simulink library "speedgoatlib_mscp"  (R2024b)
settings: Solver=VariableStepAuto  StartTime=0.0  StopTime=10.0  RelTol=1e-3
libraries: slrealtimeethercatlib x517, simulink x316, hdlsllib x168, $bdroot x11, slrealtimeutilitieslib x1
(part 4 of 5)

== system speedgoatlib_mscp/Templates/MSCP SC2191 Read Advanced Template/Channel_07 ==
  Bus Creator : BusCreator  Inputs=6  OutDataTypeStr=Bus: MscpBus_SC2191_Channel_Advanced_Read
      settings: InheritFromInputs=off
  Vhigh : slrealtimeethercatlib/EtherCAT PDO Receive  Priority=2  sig_name=Uninitialized Block  sig_offset=144  sig_type=uint8  type_size=8  sig_dim=1  device_id=0  sample_time=0.010000
  Vhigh_Gain : slrealtimeethercatlib/EtherCAT PDO Receive  Priority=2  sig_name=Uninitialized Block  sig_offset=144  sig_type=uint8  type_size=8  sig_dim=1  device_id=0  sample_time=0.010000
  Vhigh_Offset : slrealtimeethercatlib/EtherCAT PDO Receive  Priority=2  sig_name=Uninitialized Block  sig_offset=144  sig_type=uint8  type_size=8  sig_dim=1  device_id=0  sample_time=0.010000
  Vlow : slrealtimeethercatlib/EtherCAT PDO Receive  Priority=2  sig_name=Uninitialized Block  sig_offset=144  sig_type=uint8  type_size=8  sig_dim=1  device_id=0  sample_time=0.010000
  Vlow_Gain : slrealtimeethercatlib/EtherCAT PDO Receive  Priority=2  sig_name=Uninitialized Block  sig_offset=144  sig_type=uint8  type_size=8  sig_dim=1  device_id=0  sample_time=0.010000
  Vlow_Offset : slrealtimeethercatlib/EtherCAT PDO Receive  Priority=2  sig_name=Uninitialized Block  sig_offset=144  sig_type=uint8  type_size=8  sig_dim=1  device_id=0  sample_time=0.010000
  Out1 : Outport
  wires:
  Vhigh/1 -> Bus Creator/2
  Vlow/1 -> Bus Creator/1
  Bus Creator/1 -> Out1/1
  Vlow_Offset/1 -> Bus Creator/3
  Vlow_Gain/1 -> Bus Creator/4
  Vhigh_Offset/1 -> Bus Creator/5
  Vhigh_Gain/1 -> Bus Creator/6

== system speedgoatlib_mscp/Templates/MSCP SC2191 Read Advanced Template/Channel_08 ==
  Bus Creator : BusCreator  Inputs=6  OutDataTypeStr=Bus: MscpBus_SC2191_Channel_Advanced_Read
      settings: InheritFromInputs=off
  Vhigh : slrealtimeethercatlib/EtherCAT PDO Receive  Priority=2  sig_name=Uninitialized Block  sig_offset=144  sig_type=uint8  type_size=8  sig_dim=1  device_id=0  sample_time=0.010000
  Vhigh_Gain : slrealtimeethercatlib/EtherCAT PDO Receive  Priority=2  sig_name=Uninitialized Block  sig_offset=144  sig_type=uint8  type_size=8  sig_dim=1  device_id=0  sample_time=0.010000
  Vhigh_Offset : slrealtimeethercatlib/EtherCAT PDO Receive  Priority=2  sig_name=Uninitialized Block  sig_offset=144  sig_type=uint8  type_size=8  sig_dim=1  device_id=0  sample_time=0.010000
  Vlow : slrealtimeethercatlib/EtherCAT PDO Receive  Priority=2  sig_name=Uninitialized Block  sig_offset=144  sig_type=uint8  type_size=8  sig_dim=1  device_id=0  sample_time=0.010000
  Vlow_Gain : slrealtimeethercatlib/EtherCAT PDO Receive  Priority=2  sig_name=Uninitialized Block  sig_offset=144  sig_type=uint8  type_size=8  sig_dim=1  device_id=0  sample_time=0.010000
  Vlow_Offset : slrealtimeethercatlib/EtherCAT PDO Receive  Priority=2  sig_name=Uninitialized Block  sig_offset=144  sig_type=uint8  type_size=8  sig_dim=1  device_id=0  sample_time=0.010000
  Out1 : Outport
  wires:
  Vhigh_Gain/1 -> Bus Creator/6
  Vhigh_Offset/1 -> Bus Creator/5
  Vlow_Gain/1 -> Bus Creator/4
  Vlow_Offset/1 -> Bus Creator/3
  Bus Creator/1 -> Out1/1
  Vlow/1 -> Bus Creator/1
  Vhigh/1 -> Bus Creator/2

== system speedgoatlib_mscp/Templates/MSCP SC2191 Read Advanced Template/Channel_09 ==
  Bus Creator : BusCreator  Inputs=6  OutDataTypeStr=Bus: MscpBus_SC2191_Channel_Advanced_Read
      settings: InheritFromInputs=off
  Vhigh : slrealtimeethercatlib/EtherCAT PDO Receive  Priority=2  sig_name=Uninitialized Block  sig_offset=144  sig_type=uint8  type_size=8  sig_dim=1  device_id=0  sample_time=0.010000
  Vhigh_Gain : slrealtimeethercatlib/EtherCAT PDO Receive  Priority=2  sig_name=Uninitialized Block  sig_offset=144  sig_type=uint8  type_size=8  sig_dim=1  device_id=0  sample_time=0.010000
  Vhigh_Offset : slrealtimeethercatlib/EtherCAT PDO Receive  Priority=2  sig_name=Uninitialized Block  sig_offset=144  sig_type=uint8  type_size=8  sig_dim=1  device_id=0  sample_time=0.010000
  Vlow : slrealtimeethercatlib/EtherCAT PDO Receive  Priority=2  sig_name=Uninitialized Block  sig_offset=144  sig_type=uint8  type_size=8  sig_dim=1  device_id=0  sample_time=0.010000
  Vlow_Gain : slrealtimeethercatlib/EtherCAT PDO Receive  Priority=2  sig_name=Uninitialized Block  sig_offset=144  sig_type=uint8  type_size=8  sig_dim=1  device_id=0  sample_time=0.010000
  Vlow_Offset : slrealtimeethercatlib/EtherCAT PDO Receive  Priority=2  sig_name=Uninitialized Block  sig_offset=144  sig_type=uint8  type_size=8  sig_dim=1  device_id=0  sample_time=0.010000
  Out1 : Outport
  wires:
  Vhigh/1 -> Bus Creator/2
  Vlow/1 -> Bus Creator/1
  Bus Creator/1 -> Out1/1
  Vlow_Offset/1 -> Bus Creator/3
  Vlow_Gain/1 -> Bus Creator/4
  Vhigh_Offset/1 -> Bus Creator/5
  Vhigh_Gain/1 -> Bus Creator/6

== system speedgoatlib_mscp/Templates/MSCP SC2191 Read Advanced Template/Channel_10 ==
  Bus Creator : BusCreator  Inputs=6  OutDataTypeStr=Bus: MscpBus_SC2191_Channel_Advanced_Read
      settings: InheritFromInputs=off
  Vhigh : slrealtimeethercatlib/EtherCAT PDO Receive  Priority=2  sig_name=Uninitialized Block  sig_offset=144  sig_type=uint8  type_size=8  sig_dim=1  device_id=0  sample_time=0.010000
  Vhigh_Gain : slrealtimeethercatlib/EtherCAT PDO Receive  Priority=2  sig_name=Uninitialized Block  sig_offset=144  sig_type=uint8  type_size=8  sig_dim=1  device_id=0  sample_time=0.010000
  Vhigh_Offset : slrealtimeethercatlib/EtherCAT PDO Receive  Priority=2  sig_name=Uninitialized Block  sig_offset=144  sig_type=uint8  type_size=8  sig_dim=1  device_id=0  sample_time=0.010000
  Vlow : slrealtimeethercatlib/EtherCAT PDO Receive  Priority=2  sig_name=Uninitialized Block  sig_offset=144  sig_type=uint8  type_size=8  sig_dim=1  device_id=0  sample_time=0.010000
  Vlow_Gain : slrealtimeethercatlib/EtherCAT PDO Receive  Priority=2  sig_name=Uninitialized Block  sig_offset=144  sig_type=uint8  type_size=8  sig_dim=1  device_id=0  sample_time=0.010000
  Vlow_Offset : slrealtimeethercatlib/EtherCAT PDO Receive  Priority=2  sig_name=Uninitialized Block  sig_offset=144  sig_type=uint8  type_size=8  sig_dim=1  device_id=0  sample_time=0.010000
  Out1 : Outport
  wires:
  Vhigh_Gain/1 -> Bus Creator/6
  Vhigh_Offset/1 -> Bus Creator/5
  Vlow_Gain/1 -> Bus Creator/4
  Vlow_Offset/1 -> Bus Creator/3
  Bus Creator/1 -> Out1/1
  Vlow/1 -> Bus Creator/1
  Vhigh/1 -> Bus Creator/2

== system speedgoatlib_mscp/Templates/MSCP SC2191 Read Advanced Template/Channel_11 ==
  Bus Creator : BusCreator  Inputs=6  OutDataTypeStr=Bus: MscpBus_SC2191_Channel_Advanced_Read
      settings: InheritFromInputs=off
  Vhigh : slrealtimeethercatlib/EtherCAT PDO Receive  Priority=2  sig_name=Uninitialized Block  sig_offset=144  sig_type=uint8  type_size=8  sig_dim=1  device_id=0  sample_time=0.010000
  Vhigh_Gain : slrealtimeethercatlib/EtherCAT PDO Receive  Priority=2  sig_name=Uninitialized Block  sig_offset=144  sig_type=uint8  type_size=8  sig_dim=1  device_id=0  sample_time=0.010000
  Vhigh_Offset : slrealtimeethercatlib/EtherCAT PDO Receive  Priority=2  sig_name=Uninitialized Block  sig_offset=144  sig_type=uint8  type_size=8  sig_dim=1  device_id=0  sample_time=0.010000
  Vlow : slrealtimeethercatlib/EtherCAT PDO Receive  Priority=2  sig_name=Uninitialized Block  sig_offset=144  sig_type=uint8  type_size=8  sig_dim=1  device_id=0  sample_time=0.010000
  Vlow_Gain : slrealtimeethercatlib/EtherCAT PDO Receive  Priority=2  sig_name=Uninitialized Block  sig_offset=144  sig_type=uint8  type_size=8  sig_dim=1  device_id=0  sample_time=0.010000
  Vlow_Offset : slrealtimeethercatlib/EtherCAT PDO Receive  Priority=2  sig_name=Uninitialized Block  sig_offset=144  sig_type=uint8  type_size=8  sig_dim=1  device_id=0  sample_time=0.010000
  Out1 : Outport
  wires:
  Vhigh/1 -> Bus Creator/2
  Vlow/1 -> Bus Creator/1
  Bus Creator/1 -> Out1/1
  Vlow_Offset/1 -> Bus Creator/3
  Vlow_Gain/1 -> Bus Creator/4
  Vhigh_Offset/1 -> Bus Creator/5
  Vhigh_Gain/1 -> Bus Creator/6

== system speedgoatlib_mscp/Templates/MSCP SC2191 Read Advanced Template/Channel_12 ==
  Bus Creator : BusCreator  Inputs=6  OutDataTypeStr=Bus: MscpBus_SC2191_Channel_Advanced_Read
      settings: InheritFromInputs=off
  Vhigh : slrealtimeethercatlib/EtherCAT PDO Receive  Priority=2  sig_name=Uninitialized Block  sig_offset=144  sig_type=uint8  type_size=8  sig_dim=1  device_id=0  sample_time=0.010000
  Vhigh_Gain : slrealtimeethercatlib/EtherCAT PDO Receive  Priority=2  sig_name=Uninitialized Block  sig_offset=144  sig_type=uint8  type_size=8  sig_dim=1  device_id=0  sample_time=0.010000
  Vhigh_Offset : slrealtimeethercatlib/EtherCAT PDO Receive  Priority=2  sig_name=Uninitialized Block  sig_offset=144  sig_type=uint8  type_size=8  sig_dim=1  device_id=0  sample_time=0.010000
  Vlow : slrealtimeethercatlib/EtherCAT PDO Receive  Priority=2  sig_name=Uninitialized Block  sig_offset=144  sig_type=uint8  type_size=8  sig_dim=1  device_id=0  sample_time=0.010000
  Vlow_Gain : slrealtimeethercatlib/EtherCAT PDO Receive  Priority=2  sig_name=Uninitialized Block  sig_offset=144  sig_type=uint8  type_size=8  sig_dim=1  device_id=0  sample_time=0.010000
  Vlow_Offset : slrealtimeethercatlib/EtherCAT PDO Receive  Priority=2  sig_name=Uninitialized Block  sig_offset=144  sig_type=uint8  type_size=8  sig_dim=1  device_id=0  sample_time=0.010000
  Out1 : Outport
  wires:
  Vhigh_Gain/1 -> Bus Creator/6
  Vhigh_Offset/1 -> Bus Creator/5
  Vlow_Gain/1 -> Bus Creator/4
  Vlow_Offset/1 -> Bus Creator/3
  Bus Creator/1 -> Out1/1
  Vlow/1 -> Bus Creator/1
  Vhigh/1 -> Bus Creator/2

== system speedgoatlib_mscp/Templates/MSCP SC2191 Read Advanced Template/Channel_13 ==
  Bus Creator : BusCreator  Inputs=6  OutDataTypeStr=Bus: MscpBus_SC2191_Channel_Advanced_Read
      settings: InheritFromInputs=off
  Vhigh : slrealtimeethercatlib/EtherCAT PDO Receive  Priority=2  sig_name=Uninitialized Block  sig_offset=144  sig_type=uint8  type_size=8  sig_dim=1  device_id=0  sample_time=0.010000
  Vhigh_Gain : slrealtimeethercatlib/EtherCAT PDO Receive  Priority=2  sig_name=Uninitialized Block  sig_offset=144  sig_type=uint8  type_size=8  sig_dim=1  device_id=0  sample_time=0.010000
  Vhigh_Offset : slrealtimeethercatlib/EtherCAT PDO Receive  Priority=2  sig_name=Uninitialized Block  sig_offset=144  sig_type=uint8  type_size=8  sig_dim=1  device_id=0  sample_time=0.010000
  Vlow : slrealtimeethercatlib/EtherCAT PDO Receive  Priority=2  sig_name=Uninitialized Block  sig_offset=144  sig_type=uint8  type_size=8  sig_dim=1  device_id=0  sample_time=0.010000
  Vlow_Gain : slrealtimeethercatlib/EtherCAT PDO Receive  Priority=2  sig_name=Uninitialized Block  sig_offset=144  sig_type=uint8  type_size=8  sig_dim=1  device_id=0  sample_time=0.010000
  Vlow_Offset : slrealtimeethercatlib/EtherCAT PDO Receive  Priority=2  sig_name=Uninitialized Block  sig_offset=144  sig_type=uint8  type_size=8  sig_dim=1  device_id=0  sample_time=0.010000
  Out1 : Outport
  wires:
  Vhigh/1 -> Bus Creator/2
  Vlow/1 -> Bus Creator/1
  Bus Creator/1 -> Out1/1
  Vlow_Offset/1 -> Bus Creator/3
  Vlow_Gain/1 -> Bus Creator/4
  Vhigh_Offset/1 -> Bus Creator/5
  Vhigh_Gain/1 -> Bus Creator/6

== system speedgoatlib_mscp/Templates/MSCP SC2191 Read Advanced Template/Channel_14 ==
  Bus Creator : BusCreator  Inputs=6  OutDataTypeStr=Bus: MscpBus_SC2191_Channel_Advanced_Read
      settings: InheritFromInputs=off
  Vhigh : slrealtimeethercatlib/EtherCAT PDO Receive  Priority=2  sig_name=Uninitialized Block  sig_offset=144  sig_type=uint8  type_size=8  sig_dim=1  device_id=0  sample_time=0.010000
  Vhigh_Gain : slrealtimeethercatlib/EtherCAT PDO Receive  Priority=2  sig_name=Uninitialized Block  sig_offset=144  sig_type=uint8  type_size=8  sig_dim=1  device_id=0  sample_time=0.010000
  Vhigh_Offset : slrealtimeethercatlib/EtherCAT PDO Receive  Priority=2  sig_name=Uninitialized Block  sig_offset=144  sig_type=uint8  type_size=8  sig_dim=1  device_id=0  sample_time=0.010000
  Vlow : slrealtimeethercatlib/EtherCAT PDO Receive  Priority=2  sig_name=Uninitialized Block  sig_offset=144  sig_type=uint8  type_size=8  sig_dim=1  device_id=0  sample_time=0.010000
  Vlow_Gain : slrealtimeethercatlib/EtherCAT PDO Receive  Priority=2  sig_name=Uninitialized Block  sig_offset=144  sig_type=uint8  type_size=8  sig_dim=1  device_id=0  sample_time=0.010000
  Vlow_Offset : slrealtimeethercatlib/EtherCAT PDO Receive  Priority=2  sig_name=Uninitialized Block  sig_offset=144  sig_type=uint8  type_size=8  sig_dim=1  device_id=0  sample_time=0.010000
  Out1 : Outport
  wires:
  Vhigh_Gain/1 -> Bus Creator/6
  Vhigh_Offset/1 -> Bus Creator/5
  Vlow_Gain/1 -> Bus Creator/4
  Vlow_Offset/1 -> Bus Creator/3
  Bus Creator/1 -> Out1/1
  Vlow/1 -> Bus Creator/1
  Vhigh/1 -> Bus Creator/2

== system speedgoatlib_mscp/Templates/MSCP SC2191 Read Advanced Template/Channel_15 ==
  Bus Creator : BusCreator  Inputs=6  OutDataTypeStr=Bus: MscpBus_SC2191_Channel_Advanced_Read
      settings: InheritFromInputs=off
  Vhigh : slrealtimeethercatlib/EtherCAT PDO Receive  Priority=2  sig_name=Uninitialized Block  sig_offset=144  sig_type=uint8  type_size=8  sig_dim=1  device_id=0  sample_time=0.010000
  Vhigh_Gain : slrealtimeethercatlib/EtherCAT PDO Receive  Priority=2  sig_name=Uninitialized Block  sig_offset=144  sig_type=uint8  type_size=8  sig_dim=1  device_id=0  sample_time=0.010000
  Vhigh_Offset : slrealtimeethercatlib/EtherCAT PDO Receive  Priority=2  sig_name=Uninitialized Block  sig_offset=144  sig_type=uint8  type_size=8  sig_dim=1  device_id=0  sample_time=0.010000
  Vlow : slrealtimeethercatlib/EtherCAT PDO Receive  Priority=2  sig_name=Uninitialized Block  sig_offset=144  sig_type=uint8  type_size=8  sig_dim=1  device_id=0  sample_time=0.010000
  Vlow_Gain : slrealtimeethercatlib/EtherCAT PDO Receive  Priority=2  sig_name=Uninitialized Block  sig_offset=144  sig_type=uint8  type_size=8  sig_dim=1  device_id=0  sample_time=0.010000
  Vlow_Offset : slrealtimeethercatlib/EtherCAT PDO Receive  Priority=2  sig_name=Uninitialized Block  sig_offset=144  sig_type=uint8  type_size=8  sig_dim=1  device_id=0  sample_time=0.010000
  Out1 : Outport
  wires:
  Vhigh/1 -> Bus Creator/2
  Vlow/1 -> Bus Creator/1
  Bus Creator/1 -> Out1/1
  Vlow_Offset/1 -> Bus Creator/3
  Vlow_Gain/1 -> Bus Creator/4
  Vhigh_Offset/1 -> Bus Creator/5
  Vhigh_Gain/1 -> Bus Creator/6

== system speedgoatlib_mscp/Templates/MSCP SC2191 Read Advanced Template/Channel_16 ==
  Bus Creator : BusCreator  Inputs=6  OutDataTypeStr=Bus: MscpBus_SC2191_Channel_Advanced_Read
      settings: InheritFromInputs=off
  Vhigh : slrealtimeethercatlib/EtherCAT PDO Receive  Priority=2  sig_name=Uninitialized Block  sig_offset=144  sig_type=uint8  type_size=8  sig_dim=1  device_id=0  sample_time=0.010000
  Vhigh_Gain : slrealtimeethercatlib/EtherCAT PDO Receive  Priority=2  sig_name=Uninitialized Block  sig_offset=144  sig_type=uint8  type_size=8  sig_dim=1  device_id=0  sample_time=0.010000
  Vhigh_Offset : slrealtimeethercatlib/EtherCAT PDO Receive  Priority=2  sig_name=Uninitialized Block  sig_offset=144  sig_type=uint8  type_size=8  sig_dim=1  device_id=0  sample_time=0.010000
  Vlow : slrealtimeethercatlib/EtherCAT PDO Receive  Priority=2  sig_name=Uninitialized Block  sig_offset=144  sig_type=uint8  type_size=8  sig_dim=1  device_id=0  sample_time=0.010000
  Vlow_Gain : slrealtimeethercatlib/EtherCAT PDO Receive  Priority=2  sig_name=Uninitialized Block  sig_offset=144  sig_type=uint8  type_size=8  sig_dim=1  device_id=0  sample_time=0.010000
  Vlow_Offset : slrealtimeethercatlib/EtherCAT PDO Receive  Priority=2  sig_name=Uninitialized Block  sig_offset=144  sig_type=uint8  type_size=8  sig_dim=1  device_id=0  sample_time=0.010000
  Out1 : Outport
  wires:
  Vhigh_Gain/1 -> Bus Creator/6
  Vhigh_Offset/1 -> Bus Creator/5
  Vlow_Gain/1 -> Bus Creator/4
  Vlow_Offset/1 -> Bus Creator/3
  Bus Creator/1 -> Out1/1
  Vlow/1 -> Bus Creator/1
  Vhigh/1 -> Bus Creator/2

== system speedgoatlib_mscp/Templates/MSCP SC2191 Read Template/Channel_01 ==
  Bus Creator : BusCreator  Inputs=2  OutDataTypeStr=Bus: MscpBus_SC2191_Channel_Read
      settings: InheritFromInputs=off
  Vhigh : slrealtimeethercatlib/EtherCAT PDO Receive  Priority=2  sig_name=Uninitialized Block  sig_offset=144  sig_type=uint8  type_size=8  sig_dim=1  device_id=0  sample_time=0.010000
  Vlow : slrealtimeethercatlib/EtherCAT PDO Receive  Priority=2  sig_name=Uninitialized Block  sig_offset=144  sig_type=uint8  type_size=8  sig_dim=1  device_id=0  sample_time=0.010000
  Out1 : Outport
  wires:
  Bus Creator/1 -> Out1/1
  Vlow/1 -> Bus Creator/1
  Vhigh/1 -> Bus Creator/2

== system speedgoatlib_mscp/Templates/MSCP SC2191 Read Template/Channel_02 ==
  Bus Creator : BusCreator  Inputs=2  OutDataTypeStr=Bus: MscpBus_SC2191_Channel_Read
      settings: InheritFromInputs=off
  Vhigh : slrealtimeethercatlib/EtherCAT PDO Receive  Priority=2  sig_name=Uninitialized Block  sig_offset=144  sig_type=uint8  type_size=8  sig_dim=1  device_id=0  sample_time=0.010000
  Vlow : slrealtimeethercatlib/EtherCAT PDO Receive  Priority=2  sig_name=Uninitialized Block  sig_offset=144  sig_type=uint8  type_size=8  sig_dim=1  device_id=0  sample_time=0.010000
  Out1 : Outport
  wires:
  Vhigh/1 -> Bus Creator/2
  Vlow/1 -> Bus Creator/1
  Bus Creator/1 -> Out1/1

== system speedgoatlib_mscp/Templates/MSCP SC2191 Read Template/Channel_03 ==
  Bus Creator : BusCreator  Inputs=2  OutDataTypeStr=Bus: MscpBus_SC2191_Channel_Read
      settings: InheritFromInputs=off
  Vhigh : slrealtimeethercatlib/EtherCAT PDO Receive  Priority=2  sig_name=Uninitialized Block  sig_offset=144  sig_type=uint8  type_size=8  sig_dim=1  device_id=0  sample_time=0.010000
  Vlow : slrealtimeethercatlib/EtherCAT PDO Receive  Priority=2  sig_name=Uninitialized Block  sig_offset=144  sig_type=uint8  type_size=8  sig_dim=1  device_id=0  sample_time=0.010000
  Out1 : Outport
  wires:
  Bus Creator/1 -> Out1/1
  Vlow/1 -> Bus Creator/1
  Vhigh/1 -> Bus Creator/2

== system speedgoatlib_mscp/Templates/MSCP SC2191 Read Template/Channel_04 ==
  Bus Creator : BusCreator  Inputs=2  OutDataTypeStr=Bus: MscpBus_SC2191_Channel_Read
      settings: InheritFromInputs=off
  Vhigh : slrealtimeethercatlib/EtherCAT PDO Receive  Priority=2  sig_name=Uninitialized Block  sig_offset=144  sig_type=uint8  type_size=8  sig_dim=1  device_id=0  sample_time=0.010000
  Vlow : slrealtimeethercatlib/EtherCAT PDO Receive  Priority=2  sig_name=Uninitialized Block  sig_offset=144  sig_type=uint8  type_size=8  sig_dim=1  device_id=0  sample_time=0.010000
  Out1 : Outport
  wires:
  Vhigh/1 -> Bus Creator/2
  Vlow/1 -> Bus Creator/1
  Bus Creator/1 -> Out1/1

== system speedgoatlib_mscp/Templates/MSCP SC2191 Read Template/Channel_05 ==
  Bus Creator : BusCreator  Inputs=2  OutDataTypeStr=Bus: MscpBus_SC2191_Channel_Read
      settings: InheritFromInputs=off
  Vhigh : slrealtimeethercatlib/EtherCAT PDO Receive  Priority=2  sig_name=Uninitialized Block  sig_offset=144  sig_type=uint8  type_size=8  sig_dim=1  device_id=0  sample_time=0.010000
  Vlow : slrealtimeethercatlib/EtherCAT PDO Receive  Priority=2  sig_name=Uninitialized Block  sig_offset=144  sig_type=uint8  type_size=8  sig_dim=1  device_id=0  sample_time=0.010000
  Out1 : Outport
  wires:
  Bus Creator/1 -> Out1/1
  Vlow/1 -> Bus Creator/1
  Vhigh/1 -> Bus Creator/2

== system speedgoatlib_mscp/Templates/MSCP SC2191 Read Template/Channel_06 ==
  Bus Creator : BusCreator  Inputs=2  OutDataTypeStr=Bus: MscpBus_SC2191_Channel_Read
      settings: InheritFromInputs=off
  Vhigh : slrealtimeethercatlib/EtherCAT PDO Receive  Priority=2  sig_name=Uninitialized Block  sig_offset=144  sig_type=uint8  type_size=8  sig_dim=1  device_id=0  sample_time=0.010000
  Vlow : slrealtimeethercatlib/EtherCAT PDO Receive  Priority=2  sig_name=Uninitialized Block  sig_offset=144  sig_type=uint8  type_size=8  sig_dim=1  device_id=0  sample_time=0.010000
  Out1 : Outport
  wires:
  Vhigh/1 -> Bus Creator/2
  Vlow/1 -> Bus Creator/1
  Bus Creator/1 -> Out1/1

== system speedgoatlib_mscp/Templates/MSCP SC2191 Read Template/Channel_07 ==
  Bus Creator : BusCreator  Inputs=2  OutDataTypeStr=Bus: MscpBus_SC2191_Channel_Read
      settings: InheritFromInputs=off
  Vhigh : slrealtimeethercatlib/EtherCAT PDO Receive  Priority=2  sig_name=Uninitialized Block  sig_offset=144  sig_type=uint8  type_size=8  sig_dim=1  device_id=0  sample_time=0.010000
  Vlow : slrealtimeethercatlib/EtherCAT PDO Receive  Priority=2  sig_name=Uninitialized Block  sig_offset=144  sig_type=uint8  type_size=8  sig_dim=1  device_id=0  sample_time=0.010000
  Out1 : Outport
  wires:
  Bus Creator/1 -> Out1/1
  Vlow/1 -> Bus Creator/1
  Vhigh/1 -> Bus Creator/2

== system speedgoatlib_mscp/Templates/MSCP SC2191 Read Template/Channel_08 ==
  Bus Creator : BusCreator  Inputs=2  OutDataTypeStr=Bus: MscpBus_SC2191_Channel_Read
      settings: InheritFromInputs=off
  Vhigh : slrealtimeethercatlib/EtherCAT PDO Receive  Priority=2  sig_name=Uninitialized Block  sig_offset=144  sig_type=uint8  type_size=8  sig_dim=1  device_id=0  sample_time=0.010000
  Vlow : slrealtimeethercatlib/EtherCAT PDO Receive  Priority=2  sig_name=Uninitialized Block  sig_offset=144  sig_type=uint8  type_size=8  sig_dim=1  device_id=0  sample_time=0.010000
  Out1 : Outport
  wires:
  Vhigh/1 -> Bus Creator/2
  Vlow/1 -> Bus Creator/1
  Bus Creator/1 -> Out1/1

== system speedgoatlib_mscp/Templates/MSCP SC2191 Read Template/Channel_09 ==
  Bus Creator : BusCreator  Inputs=2  OutDataTypeStr=Bus: MscpBus_SC2191_Channel_Read
      settings: InheritFromInputs=off
  Vhigh : slrealtimeethercatlib/EtherCAT PDO Receive  Priority=2  sig_name=Uninitialized Block  sig_offset=144  sig_type=uint8  type_size=8  sig_dim=1  device_id=0  sample_time=0.010000
  Vlow : slrealtimeethercatlib/EtherCAT PDO Receive  Priority=2  sig_name=Uninitialized Block  sig_offset=144  sig_type=uint8  type_size=8  sig_dim=1  device_id=0  sample_time=0.010000
  Out1 : Outport
  wires:
  Bus Creator/1 -> Out1/1
  Vlow/1 -> Bus Creator/1
  Vhigh/1 -> Bus Creator/2

== system speedgoatlib_mscp/Templates/MSCP SC2191 Read Template/Channel_10 ==
  Bus Creator : BusCreator  Inputs=2  OutDataTypeStr=Bus: MscpBus_SC2191_Channel_Read
      settings: InheritFromInputs=off
  Vhigh : slrealtimeethercatlib/EtherCAT PDO Receive  Priority=2  sig_name=Uninitialized Block  sig_offset=144  sig_type=uint8  type_size=8  sig_dim=1  device_id=0  sample_time=0.010000
  Vlow : slrealtimeethercatlib/EtherCAT PDO Receive  Priority=2  sig_name=Uninitialized Block  sig_offset=144  sig_type=uint8  type_size=8  sig_dim=1  device_id=0  sample_time=0.010000
  Out1 : Outport
  wires:
  Vhigh/1 -> Bus Creator/2
  Vlow/1 -> Bus Creator/1
  Bus Creator/1 -> Out1/1

== system speedgoatlib_mscp/Templates/MSCP SC2191 Read Template/Channel_11 ==
  Bus Creator : BusCreator  Inputs=2  OutDataTypeStr=Bus: MscpBus_SC2191_Channel_Read
      settings: InheritFromInputs=off
  Vhigh : slrealtimeethercatlib/EtherCAT PDO Receive  Priority=2  sig_name=Uninitialized Block  sig_offset=144  sig_type=uint8  type_size=8  sig_dim=1  device_id=0  sample_time=0.010000
  Vlow : slrealtimeethercatlib/EtherCAT PDO Receive  Priority=2  sig_name=Uninitialized Block  sig_offset=144  sig_type=uint8  type_size=8  sig_dim=1  device_id=0  sample_time=0.010000
  Out1 : Outport
  wires:
  Bus Creator/1 -> Out1/1
  Vlow/1 -> Bus Creator/1
  Vhigh/1 -> Bus Creator/2

== system speedgoatlib_mscp/Templates/MSCP SC2191 Read Template/Channel_12 ==
  Bus Creator : BusCreator  Inputs=2  OutDataTypeStr=Bus: MscpBus_SC2191_Channel_Read
      settings: InheritFromInputs=off
  Vhigh : slrealtimeethercatlib/EtherCAT PDO Receive  Priority=2  sig_name=Uninitialized Block  sig_offset=144  sig_type=uint8  type_size=8  sig_dim=1  device_id=0  sample_time=0.010000
  Vlow : slrealtimeethercatlib/EtherCAT PDO Receive  Priority=2  sig_name=Uninitialized Block  sig_offset=144  sig_type=uint8  type_size=8  sig_dim=1  device_id=0  sample_time=0.010000
  Out1 : Outport
  wires:
  Vhigh/1 -> Bus Creator/2
  Vlow/1 -> Bus Creator/1
  Bus Creator/1 -> Out1/1

== system speedgoatlib_mscp/Templates/MSCP SC2191 Read Template/Channel_13 ==
  Bus Creator : BusCreator  Inputs=2  OutDataTypeStr=Bus: MscpBus_SC2191_Channel_Read
      settings: InheritFromInputs=off
  Vhigh : slrealtimeethercatlib/EtherCAT PDO Receive  Priority=2  sig_name=Uninitialized Block  sig_offset=144  sig_type=uint8  type_size=8  sig_dim=1  device_id=0  sample_time=0.010000
  Vlow : slrealtimeethercatlib/EtherCAT PDO Receive  Priority=2  sig_name=Uninitialized Block  sig_offset=144  sig_type=uint8  type_size=8  sig_dim=1  device_id=0  sample_time=0.010000
  Out1 : Outport
  wires:
  Bus Creator/1 -> Out1/1
  Vlow/1 -> Bus Creator/1
  Vhigh/1 -> Bus Creator/2

== system speedgoatlib_mscp/Templates/MSCP SC2191 Read Template/Channel_14 ==
  Bus Creator : BusCreator  Inputs=2  OutDataTypeStr=Bus: MscpBus_SC2191_Channel_Read
      settings: InheritFromInputs=off
  Vhigh : slrealtimeethercatlib/EtherCAT PDO Receive  Priority=2  sig_name=Uninitialized Block  sig_offset=144  sig_type=uint8  type_size=8  sig_dim=1  device_id=0  sample_time=0.010000
  Vlow : slrealtimeethercatlib/EtherCAT PDO Receive  Priority=2  sig_name=Uninitialized Block  sig_offset=144  sig_type=uint8  type_size=8  sig_dim=1  device_id=0  sample_time=0.010000
  Out1 : Outport
  wires:
  Vhigh/1 -> Bus Creator/2
  Vlow/1 -> Bus Creator/1
  Bus Creator/1 -> Out1/1

== system speedgoatlib_mscp/Templates/MSCP SC2191 Read Template/Channel_15 ==
  Bus Creator : BusCreator  Inputs=2  OutDataTypeStr=Bus: MscpBus_SC2191_Channel_Read
      settings: InheritFromInputs=off
  Vhigh : slrealtimeethercatlib/EtherCAT PDO Receive  Priority=2  sig_name=Uninitialized Block  sig_offset=144  sig_type=uint8  type_size=8  sig_dim=1  device_id=0  sample_time=0.010000
  Vlow : slrealtimeethercatlib/EtherCAT PDO Receive  Priority=2  sig_name=Uninitialized Block  sig_offset=144  sig_type=uint8  type_size=8  sig_dim=1  device_id=0  sample_time=0.010000
  Out1 : Outport
  wires:
  Bus Creator/1 -> Out1/1
  Vlow/1 -> Bus Creator/1
  Vhigh/1 -> Bus Creator/2

== system speedgoatlib_mscp/Templates/MSCP SC2191 Read Template/Channel_16 ==
  Bus Creator : BusCreator  Inputs=2  OutDataTypeStr=Bus: MscpBus_SC2191_Channel_Read
      settings: InheritFromInputs=off
  Vhigh : slrealtimeethercatlib/EtherCAT PDO Receive  Priority=2  sig_name=Uninitialized Block  sig_offset=144  sig_type=uint8  type_size=8  sig_dim=1  device_id=0  sample_time=0.010000
  Vlow : slrealtimeethercatlib/EtherCAT PDO Receive  Priority=2  sig_name=Uninitialized Block  sig_offset=144  sig_type=uint8  type_size=8  sig_dim=1  device_id=0  sample_time=0.010000
  Out1 : Outport
  wires:
  Vhigh/1 -> Bus Creator/2
  Vlow/1 -> Bus Creator/1
  Bus Creator/1 -> Out1/1

== system speedgoatlib_mscp/Templates/MSCP SC2191 Write Advanced Template/Channel_01 ==
  In1 : Inport  OutDataTypeStr=Bus: MscpBus_SC2191_Channel_Advanced_Write
  Bus Selector : BusSelector  OutputSignals=Configuration,Vlow,Vhigh,Enable_Correction_Values,Vlow_Offset,Vlow_Gain,Vhigh_Offset,Vhigh_Gain
  Configuration : slrealtimeethercatlib/EtherCAT PDO Transmit  Priority=3  sig_name=Uninitialized Block  sig_offset=128  sig_type=uint8  type_size=8  sig_dim=1  device_id=0  sample_time=0.010000
  Enable_Correction_Values : slrealtimeethercatlib/EtherCAT PDO Transmit  Priority=3  sig_name=Uninitialized Block  sig_offset=128  sig_type=uint8  type_size=8  sig_dim=1  device_id=0  sample_time=0.010000
  SetConfig : simulink/Logic and Bit Operations/Bitwise Operator  logicop=OR  UseBitMask=on  BitMask=0b00000000  BitMaskRealWorld=Stored Integer
      settings: LibrarySourceBlock=|
      | simulink/Quick Insert/Logic and Bit
      | Operations/Bitwise OR
  Vhigh : slrealtimeethercatlib/EtherCAT PDO Transmit  Priority=3  sig_name=Uninitialized Block  sig_offset=128  sig_type=uint8  type_size=8  sig_dim=1  device_id=0  sample_time=0.010000
  Vhigh_Gain : slrealtimeethercatlib/EtherCAT PDO Transmit  Priority=3  sig_name=Uninitialized Block  sig_offset=128  sig_type=uint8  type_size=8  sig_dim=1  device_id=0  sample_time=0.010000
  Vhigh_Offset : slrealtimeethercatlib/EtherCAT PDO Transmit  Priority=3  sig_name=Uninitialized Block  sig_offset=128  sig_type=uint8  type_size=8  sig_dim=1  device_id=0  sample_time=0.010000
  Vlow : slrealtimeethercatlib/EtherCAT PDO Transmit  Priority=3  sig_name=Uninitialized Block  sig_offset=128  sig_type=uint8  type_size=8  sig_dim=1  device_id=0  sample_time=0.010000
  Vlow_Gain : slrealtimeethercatlib/EtherCAT PDO Transmit  Priority=3  sig_name=Uninitialized Block  sig_offset=128  sig_type=uint8  type_size=8  sig_dim=1  device_id=0  sample_time=0.010000
  Vlow_Offset : slrealtimeethercatlib/EtherCAT PDO Transmit  Priority=3  sig_name=Uninitialized Block  sig_offset=128  sig_type=uint8  type_size=8  sig_dim=1  device_id=0  sample_time=0.010000
  wires:
  In1/1 -> Bus Selector/1
  Bus Selector/1 -> SetConfig/1  "<Configuration>"
  Bus Selector/2 -> Vlow/1  "<Vlow>"
  Bus Selector/3 -> Vhigh/1  "<Vhigh>"
  Bus Selector/4 -> Enable_Correction_Values/1  "<Enable_Correction_Values>"
  Bus Selector/5 -> Vlow_Offset/1  "<Vlow_Offset>"
  Bus Selector/6 -> Vlow_Gain/1  "<Vlow_Gain>"
  Bus Selector/7 -> Vhigh_Offset/1  "<Vhigh_Offset>"
  Bus Selector/8 -> Vhigh_Gain/1  "<Vhigh_Gain>"
  SetConfig/1 -> Configuration/1

== system speedgoatlib_mscp/Templates/MSCP SC2191 Write Advanced Template/Channel_02 ==
  In1 : Inport  OutDataTypeStr=Bus: MscpBus_SC2191_Channel_Advanced_Write
  Bus Selector : BusSelector  OutputSignals=Configuration,Vlow,Vhigh,Enable_Correction_Values,Vlow_Offset,Vlow_Gain,Vhigh_Offset,Vhigh_Gain
  Configuration : slrealtimeethercatlib/EtherCAT PDO Transmit  Priority=3  sig_name=Uninitialized Block  sig_offset=128  sig_type=uint8  type_size=8  sig_dim=1  device_id=0  sample_time=0.010000
  Enable_Correction_Values : slrealtimeethercatlib/EtherCAT PDO Transmit  Priority=3  sig_name=Uninitialized Block  sig_offset=128  sig_type=uint8  type_size=8  sig_dim=1  device_id=0  sample_time=0.010000
  SetConfig : simulink/Logic and Bit Operations/Bitwise Operator  logicop=OR  UseBitMask=on  BitMask=0b00000000  BitMaskRealWorld=Stored Integer
      settings: LibrarySourceBlock=|
      | simulink/Quick Insert/Logic and Bit
      | Operations/Bitwise OR
  Vhigh : slrealtimeethercatlib/EtherCAT PDO Transmit  Priority=3  sig_name=Uninitialized Block  sig_offset=128  sig_type=uint8  type_size=8  sig_dim=1  device_id=0  sample_time=0.010000
  Vhigh_Gain : slrealtimeethercatlib/EtherCAT PDO Transmit  Priority=3  sig_name=Uninitialized Block  sig_offset=128  sig_type=uint8  type_size=8  sig_dim=1  device_id=0  sample_time=0.010000
  Vhigh_Offset : slrealtimeethercatlib/EtherCAT PDO Transmit  Priority=3  sig_name=Uninitialized Block  sig_offset=128  sig_type=uint8  type_size=8  sig_dim=1  device_id=0  sample_time=0.010000
  Vlow : slrealtimeethercatlib/EtherCAT PDO Transmit  Priority=3  sig_name=Uninitialized Block  sig_offset=128  sig_type=uint8  type_size=8  sig_dim=1  device_id=0  sample_time=0.010000
  Vlow_Gain : slrealtimeethercatlib/EtherCAT PDO Transmit  Priority=3  sig_name=Uninitialized Block  sig_offset=128  sig_type=uint8  type_size=8  sig_dim=1  device_id=0  sample_time=0.010000
  Vlow_Offset : slrealtimeethercatlib/EtherCAT PDO Transmit  Priority=3  sig_name=Uninitialized Block  sig_offset=128  sig_type=uint8  type_size=8  sig_dim=1  device_id=0  sample_time=0.010000
  wires:
  Bus Selector/8 -> Vhigh_Gain/1  "<Vhigh_Gain>"
  Bus Selector/7 -> Vhigh_Offset/1  "<Vhigh_Offset>"
  Bus Selector/6 -> Vlow_Gain/1  "<Vlow_Gain>"
  Bus Selector/5 -> Vlow_Offset/1  "<Vlow_Offset>"
  Bus Selector/4 -> Enable_Correction_Values/1  "<Enable_Correction_Values>"
  Bus Selector/3 -> Vhigh/1  "<Vhigh>"
  Bus Selector/2 -> Vlow/1  "<Vlow>"
  Bus Selector/1 -> SetConfig/1  "<Configuration>"
  In1/1 -> Bus Selector/1
  SetConfig/1 -> Configuration/1

== system speedgoatlib_mscp/Templates/MSCP SC2191 Write Advanced Template/Channel_03 ==
  In1 : Inport  OutDataTypeStr=Bus: MscpBus_SC2191_Channel_Advanced_Write
  Bus Selector : BusSelector  OutputSignals=Configuration,Vlow,Vhigh,Enable_Correction_Values,Vlow_Offset,Vlow_Gain,Vhigh_Offset,Vhigh_Gain
  Configuration : slrealtimeethercatlib/EtherCAT PDO Transmit  Priority=3  sig_name=Uninitialized Block  sig_offset=128  sig_type=uint8  type_size=8  sig_dim=1  device_id=0  sample_time=0.010000
  Enable_Correction_Values : slrealtimeethercatlib/EtherCAT PDO Transmit  Priority=3  sig_name=Uninitialized Block  sig_offset=128  sig_type=uint8  type_size=8  sig_dim=1  device_id=0  sample_time=0.010000
  SetConfig : simulink/Logic and Bit Operations/Bitwise Operator  logicop=OR  UseBitMask=on  BitMask=0b00000000  BitMaskRealWorld=Stored Integer
      settings: LibrarySourceBlock=|
      | simulink/Quick Insert/Logic and Bit
      | Operations/Bitwise OR
  Vhigh : slrealtimeethercatlib/EtherCAT PDO Transmit  Priority=3  sig_name=Uninitialized Block  sig_offset=128  sig_type=uint8  type_size=8  sig_dim=1  device_id=0  sample_time=0.010000
  Vhigh_Gain : slrealtimeethercatlib/EtherCAT PDO Transmit  Priority=3  sig_name=Uninitialized Block  sig_offset=128  sig_type=uint8  type_size=8  sig_dim=1  device_id=0  sample_time=0.010000
  Vhigh_Offset : slrealtimeethercatlib/EtherCAT PDO Transmit  Priority=3  sig_name=Uninitialized Block  sig_offset=128  sig_type=uint8  type_size=8  sig_dim=1  device_id=0  sample_time=0.010000
  Vlow : slrealtimeethercatlib/EtherCAT PDO Transmit  Priority=3  sig_name=Uninitialized Block  sig_offset=128  sig_type=uint8  type_size=8  sig_dim=1  device_id=0  sample_time=0.010000
  Vlow_Gain : slrealtimeethercatlib/EtherCAT PDO Transmit  Priority=3  sig_name=Uninitialized Block  sig_offset=128  sig_type=uint8  type_size=8  sig_dim=1  device_id=0  sample_time=0.010000
  Vlow_Offset : slrealtimeethercatlib/EtherCAT PDO Transmit  Priority=3  sig_name=Uninitialized Block  sig_offset=128  sig_type=uint8  type_size=8  sig_dim=1  device_id=0  sample_time=0.010000
  wires:
  In1/1 -> Bus Selector/1
  Bus Selector/1 -> SetConfig/1  "<Configuration>"
  Bus Selector/2 -> Vlow/1  "<Vlow>"
  Bus Selector/3 -> Vhigh/1  "<Vhigh>"
  Bus Selector/4 -> Enable_Correction_Values/1  "<Enable_Correction_Values>"
  Bus Selector/5 -> Vlow_Offset/1  "<Vlow_Offset>"
  Bus Selector/6 -> Vlow_Gain/1  "<Vlow_Gain>"
  Bus Selector/7 -> Vhigh_Offset/1  "<Vhigh_Offset>"
  Bus Selector/8 -> Vhigh_Gain/1  "<Vhigh_Gain>"
  SetConfig/1 -> Configuration/1

== system speedgoatlib_mscp/Templates/MSCP SC2191 Write Advanced Template/Channel_04 ==
  In1 : Inport  OutDataTypeStr=Bus: MscpBus_SC2191_Channel_Advanced_Write
  Bus Selector : BusSelector  OutputSignals=Configuration,Vlow,Vhigh,Enable_Correction_Values,Vlow_Offset,Vlow_Gain,Vhigh_Offset,Vhigh_Gain
  Configuration : slrealtimeethercatlib/EtherCAT PDO Transmit  Priority=3  sig_name=Uninitialized Block  sig_offset=128  sig_type=uint8  type_size=8  sig_dim=1  device_id=0  sample_time=0.010000
  Enable_Correction_Values : slrealtimeethercatlib/EtherCAT PDO Transmit  Priority=3  sig_name=Uninitialized Block  sig_offset=128  sig_type=uint8  type_size=8  sig_dim=1  device_id=0  sample_time=0.010000
  SetConfig : simulink/Logic and Bit Operations/Bitwise Operator  logicop=OR  UseBitMask=on  BitMask=0b00000000  BitMaskRealWorld=Stored Integer
      settings: LibrarySourceBlock=|
      | simulink/Quick Insert/Logic and Bit
      | Operations/Bitwise OR
  Vhigh : slrealtimeethercatlib/EtherCAT PDO Transmit  Priority=3  sig_name=Uninitialized Block  sig_offset=128  sig_type=uint8  type_size=8  sig_dim=1  device_id=0  sample_time=0.010000
  Vhigh_Gain : slrealtimeethercatlib/EtherCAT PDO Transmit  Priority=3  sig_name=Uninitialized Block  sig_offset=128  sig_type=uint8  type_size=8  sig_dim=1  device_id=0  sample_time=0.010000
  Vhigh_Offset : slrealtimeethercatlib/EtherCAT PDO Transmit  Priority=3  sig_name=Uninitialized Block  sig_offset=128  sig_type=uint8  type_size=8  sig_dim=1  device_id=0  sample_time=0.010000
  Vlow : slrealtimeethercatlib/EtherCAT PDO Transmit  Priority=3  sig_name=Uninitialized Block  sig_offset=128  sig_type=uint8  type_size=8  sig_dim=1  device_id=0  sample_time=0.010000
  Vlow_Gain : slrealtimeethercatlib/EtherCAT PDO Transmit  Priority=3  sig_name=Uninitialized Block  sig_offset=128  sig_type=uint8  type_size=8  sig_dim=1  device_id=0  sample_time=0.010000
  Vlow_Offset : slrealtimeethercatlib/EtherCAT PDO Transmit  Priority=3  sig_name=Uninitialized Block  sig_offset=128  sig_type=uint8  type_size=8  sig_dim=1  device_id=0  sample_time=0.010000
  wires:
  Bus Selector/8 -> Vhigh_Gain/1  "<Vhigh_Gain>"
  Bus Selector/7 -> Vhigh_Offset/1  "<Vhigh_Offset>"
  Bus Selector/6 -> Vlow_Gain/1  "<Vlow_Gain>"
  Bus Selector/5 -> Vlow_Offset/1  "<Vlow_Offset>"
  Bus Selector/4 -> Enable_Correction_Values/1  "<Enable_Correction_Values>"
  Bus Selector/3 -> Vhigh/1  "<Vhigh>"
  Bus Selector/2 -> Vlow/1  "<Vlow>"
  Bus Selector/1 -> SetConfig/1  "<Configuration>"
  In1/1 -> Bus Selector/1
  SetConfig/1 -> Configuration/1

== system speedgoatlib_mscp/Templates/MSCP SC2191 Write Advanced Template/Channel_05 ==
  In1 : Inport  OutDataTypeStr=Bus: MscpBus_SC2191_Channel_Advanced_Write
  Bus Selector : BusSelector  OutputSignals=Configuration,Vlow,Vhigh,Enable_Correction_Values,Vlow_Offset,Vlow_Gain,Vhigh_Offset,Vhigh_Gain
  Configuration : slrealtimeethercatlib/EtherCAT PDO Transmit  Priority=3  sig_name=Uninitialized Block  sig_offset=128  sig_type=uint8  type_size=8  sig_dim=1  device_id=0  sample_time=0.010000
  Enable_Correction_Values : slrealtimeethercatlib/EtherCAT PDO Transmit  Priority=3  sig_name=Uninitialized Block  sig_offset=128  sig_type=uint8  type_size=8  sig_dim=1  device_id=0  sample_time=0.010000
  SetConfig : simulink/Logic and Bit Operations/Bitwise Operator  logicop=OR  UseBitMask=on  BitMask=0b00000000  BitMaskRealWorld=Stored Integer
      settings: LibrarySourceBlock=|
      | simulink/Quick Insert/Logic and Bit
      | Operations/Bitwise OR
  Vhigh : slrealtimeethercatlib/EtherCAT PDO Transmit  Priority=3  sig_name=Uninitialized Block  sig_offset=128  sig_type=uint8  type_size=8  sig_dim=1  device_id=0  sample_time=0.010000
  Vhigh_Gain : slrealtimeethercatlib/EtherCAT PDO Transmit  Priority=3  sig_name=Uninitialized Block  sig_offset=128  sig_type=uint8  type_size=8  sig_dim=1  device_id=0  sample_time=0.010000
  Vhigh_Offset : slrealtimeethercatlib/EtherCAT PDO Transmit  Priority=3  sig_name=Uninitialized Block  sig_offset=128  sig_type=uint8  type_size=8  sig_dim=1  device_id=0  sample_time=0.010000
  Vlow : slrealtimeethercatlib/EtherCAT PDO Transmit  Priority=3  sig_name=Uninitialized Block  sig_offset=128  sig_type=uint8  type_size=8  sig_dim=1  device_id=0  sample_time=0.010000
  Vlow_Gain : slrealtimeethercatlib/EtherCAT PDO Transmit  Priority=3  sig_name=Uninitialized Block  sig_offset=128  sig_type=uint8  type_size=8  sig_dim=1  device_id=0  sample_time=0.010000
  Vlow_Offset : slrealtimeethercatlib/EtherCAT PDO Transmit  Priority=3  sig_name=Uninitialized Block  sig_offset=128  sig_type=uint8  type_size=8  sig_dim=1  device_id=0  sample_time=0.010000
  wires:
  In1/1 -> Bus Selector/1
  Bus Selector/1 -> SetConfig/1  "<Configuration>"
  Bus Selector/2 -> Vlow/1  "<Vlow>"
  Bus Selector/3 -> Vhigh/1  "<Vhigh>"
  Bus Selector/4 -> Enable_Correction_Values/1  "<Enable_Correction_Values>"
  Bus Selector/5 -> Vlow_Offset/1  "<Vlow_Offset>"
  Bus Selector/6 -> Vlow_Gain/1  "<Vlow_Gain>"
  Bus Selector/7 -> Vhigh_Offset/1  "<Vhigh_Offset>"
  Bus Selector/8 -> Vhigh_Gain/1  "<Vhigh_Gain>"
  SetConfig/1 -> Configuration/1

== system speedgoatlib_mscp/Templates/MSCP SC2191 Write Advanced Template/Channel_06 ==
  In1 : Inport  OutDataTypeStr=Bus: MscpBus_SC2191_Channel_Advanced_Write
  Bus Selector : BusSelector  OutputSignals=Configuration,Vlow,Vhigh,Enable_Correction_Values,Vlow_Offset,Vlow_Gain,Vhigh_Offset,Vhigh_Gain
  Configuration : slrealtimeethercatlib/EtherCAT PDO Transmit  Priority=3  sig_name=Uninitialized Block  sig_offset=128  sig_type=uint8  type_size=8  sig_dim=1  device_id=0  sample_time=0.010000
  Enable_Correction_Values : slrealtimeethercatlib/EtherCAT PDO Transmit  Priority=3  sig_name=Uninitialized Block  sig_offset=128  sig_type=uint8  type_size=8  sig_dim=1  device_id=0  sample_time=0.010000
  SetConfig : simulink/Logic and Bit Operations/Bitwise Operator  logicop=OR  UseBitMask=on  BitMask=0b00000000  BitMaskRealWorld=Stored Integer
      settings: LibrarySourceBlock=|
      | simulink/Quick Insert/Logic and Bit
      | Operations/Bitwise OR
  Vhigh : slrealtimeethercatlib/EtherCAT PDO Transmit  Priority=3  sig_name=Uninitialized Block  sig_offset=128  sig_type=uint8  type_size=8  sig_dim=1  device_id=0  sample_time=0.010000
  Vhigh_Gain : slrealtimeethercatlib/EtherCAT PDO Transmit  Priority=3  sig_name=Uninitialized Block  sig_offset=128  sig_type=uint8  type_size=8  sig_dim=1  device_id=0  sample_time=0.010000
  Vhigh_Offset : slrealtimeethercatlib/EtherCAT PDO Transmit  Priority=3  sig_name=Uninitialized Block  sig_offset=128  sig_type=uint8  type_size=8  sig_dim=1  device_id=0  sample_time=0.010000
  Vlow : slrealtimeethercatlib/EtherCAT PDO Transmit  Priority=3  sig_name=Uninitialized Block  sig_offset=128  sig_type=uint8  type_size=8  sig_dim=1  device_id=0  sample_time=0.010000
  Vlow_Gain : slrealtimeethercatlib/EtherCAT PDO Transmit  Priority=3  sig_name=Uninitialized Block  sig_offset=128  sig_type=uint8  type_size=8  sig_dim=1  device_id=0  sample_time=0.010000
  Vlow_Offset : slrealtimeethercatlib/EtherCAT PDO Transmit  Priority=3  sig_name=Uninitialized Block  sig_offset=128  sig_type=uint8  type_size=8  sig_dim=1  device_id=0  sample_time=0.010000
  wires:
  Bus Selector/8 -> Vhigh_Gain/1  "<Vhigh_Gain>"
  Bus Selector/7 -> Vhigh_Offset/1  "<Vhigh_Offset>"
  Bus Selector/6 -> Vlow_Gain/1  "<Vlow_Gain>"
  Bus Selector/5 -> Vlow_Offset/1  "<Vlow_Offset>"
  Bus Selector/4 -> Enable_Correction_Values/1  "<Enable_Correction_Values>"
  Bus Selector/3 -> Vhigh/1  "<Vhigh>"
  Bus Selector/2 -> Vlow/1  "<Vlow>"
  Bus Selector/1 -> SetConfig/1  "<Configuration>"
  In1/1 -> Bus Selector/1
  SetConfig/1 -> Configuration/1

== system speedgoatlib_mscp/Templates/MSCP SC2191 Write Advanced Template/Channel_07 ==
  In1 : Inport  OutDataTypeStr=Bus: MscpBus_SC2191_Channel_Advanced_Write
  Bus Selector : BusSelector  OutputSignals=Configuration,Vlow,Vhigh,Enable_Correction_Values,Vlow_Offset,Vlow_Gain,Vhigh_Offset,Vhigh_Gain
  Configuration : slrealtimeethercatlib/EtherCAT PDO Transmit  Priority=3  sig_name=Uninitialized Block  sig_offset=128  sig_type=uint8  type_size=8  sig_dim=1  device_id=0  sample_time=0.010000
  Enable_Correction_Values : slrealtimeethercatlib/EtherCAT PDO Transmit  Priority=3  sig_name=Uninitialized Block  sig_offset=128  sig_type=uint8  type_size=8  sig_dim=1  device_id=0  sample_time=0.010000
  SetConfig : simulink/Logic and Bit Operations/Bitwise Operator  logicop=OR  UseBitMask=on  BitMask=0b00000000  BitMaskRealWorld=Stored Integer
      settings: LibrarySourceBlock=|
      | simulink/Quick Insert/Logic and Bit
      | Operations/Bitwise OR
  Vhigh : slrealtimeethercatlib/EtherCAT PDO Transmit  Priority=3  sig_name=Uninitialized Block  sig_offset=128  sig_type=uint8  type_size=8  sig_dim=1  device_id=0  sample_time=0.010000
  Vhigh_Gain : slrealtimeethercatlib/EtherCAT PDO Transmit  Priority=3  sig_name=Uninitialized Block  sig_offset=128  sig_type=uint8  type_size=8  sig_dim=1  device_id=0  sample_time=0.010000
  Vhigh_Offset : slrealtimeethercatlib/EtherCAT PDO Transmit  Priority=3  sig_name=Uninitialized Block  sig_offset=128  sig_type=uint8  type_size=8  sig_dim=1  device_id=0  sample_time=0.010000
  Vlow : slrealtimeethercatlib/EtherCAT PDO Transmit  Priority=3  sig_name=Uninitialized Block  sig_offset=128  sig_type=uint8  type_size=8  sig_dim=1  device_id=0  sample_time=0.010000
  Vlow_Gain : slrealtimeethercatlib/EtherCAT PDO Transmit  Priority=3  sig_name=Uninitialized Block  sig_offset=128  sig_type=uint8  type_size=8  sig_dim=1  device_id=0  sample_time=0.010000
  Vlow_Offset : slrealtimeethercatlib/EtherCAT PDO Transmit  Priority=3  sig_name=Uninitialized Block  sig_offset=128  sig_type=uint8  type_size=8  sig_dim=1  device_id=0  sample_time=0.010000
  wires:
  In1/1 -> Bus Selector/1
  Bus Selector/1 -> SetConfig/1  "<Configuration>"
  Bus Selector/2 -> Vlow/1  "<Vlow>"
  Bus Selector/3 -> Vhigh/1  "<Vhigh>"
  Bus Selector/4 -> Enable_Correction_Values/1  "<Enable_Correction_Values>"
  Bus Selector/5 -> Vlow_Offset/1  "<Vlow_Offset>"
  Bus Selector/6 -> Vlow_Gain/1  "<Vlow_Gain>"
  Bus Selector/7 -> Vhigh_Offset/1  "<Vhigh_Offset>"
  Bus Selector/8 -> Vhigh_Gain/1  "<Vhigh_Gain>"
  SetConfig/1 -> Configuration/1

== system speedgoatlib_mscp/Templates/MSCP SC2191 Write Advanced Template/Channel_08 ==
  In1 : Inport  OutDataTypeStr=Bus: MscpBus_SC2191_Channel_Advanced_Write
  Bus Selector : BusSelector  OutputSignals=Configuration,Vlow,Vhigh,Enable_Correction_Values,Vlow_Offset,Vlow_Gain,Vhigh_Offset,Vhigh_Gain
  Configuration : slrealtimeethercatlib/EtherCAT PDO Transmit  Priority=3  sig_name=Uninitialized Block  sig_offset=128  sig_type=uint8  type_size=8  sig_dim=1  device_id=0  sample_time=0.010000
  Enable_Correction_Values : slrealtimeethercatlib/EtherCAT PDO Transmit  Priority=3  sig_name=Uninitialized Block  sig_offset=128  sig_type=uint8  type_size=8  sig_dim=1  device_id=0  sample_time=0.010000
  SetConfig : simulink/Logic and Bit Operations/Bitwise Operator  logicop=OR  UseBitMask=on  BitMask=0b00000000  BitMaskRealWorld=Stored Integer
      settings: LibrarySourceBlock=|
      | simulink/Quick Insert/Logic and Bit
      | Operations/Bitwise OR
  Vhigh : slrealtimeethercatlib/EtherCAT PDO Transmit  Priority=3  sig_name=Uninitialized Block  sig_offset=128  sig_type=uint8  type_size=8  sig_dim=1  device_id=0  sample_time=0.010000
  Vhigh_Gain : slrealtimeethercatlib/EtherCAT PDO Transmit  Priority=3  sig_name=Uninitialized Block  sig_offset=128  sig_type=uint8  type_size=8  sig_dim=1  device_id=0  sample_time=0.010000
  Vhigh_Offset : slrealtimeethercatlib/EtherCAT PDO Transmit  Priority=3  sig_name=Uninitialized Block  sig_offset=128  sig_type=uint8  type_size=8  sig_dim=1  device_id=0  sample_time=0.010000
  Vlow : slrealtimeethercatlib/EtherCAT PDO Transmit  Priority=3  sig_name=Uninitialized Block  sig_offset=128  sig_type=uint8  type_size=8  sig_dim=1  device_id=0  sample_time=0.010000
  Vlow_Gain : slrealtimeethercatlib/EtherCAT PDO Transmit  Priority=3  sig_name=Uninitialized Block  sig_offset=128  sig_type=uint8  type_size=8  sig_dim=1  device_id=0  sample_time=0.010000
  Vlow_Offset : slrealtimeethercatlib/EtherCAT PDO Transmit  Priority=3  sig_name=Uninitialized Block  sig_offset=128  sig_type=uint8  type_size=8  sig_dim=1  device_id=0  sample_time=0.010000
  wires:
  Bus Selector/8 -> Vhigh_Gain/1  "<Vhigh_Gain>"
  Bus Selector/7 -> Vhigh_Offset/1  "<Vhigh_Offset>"
  Bus Selector/6 -> Vlow_Gain/1  "<Vlow_Gain>"
  Bus Selector/5 -> Vlow_Offset/1  "<Vlow_Offset>"
  Bus Selector/4 -> Enable_Correction_Values/1  "<Enable_Correction_Values>"
  Bus Selector/3 -> Vhigh/1  "<Vhigh>"
  Bus Selector/2 -> Vlow/1  "<Vlow>"
  Bus Selector/1 -> SetConfig/1  "<Configuration>"
  In1/1 -> Bus Selector/1
  SetConfig/1 -> Configuration/1
